simulink model "Ex4_System_Level_AntennaArray"  (R2025b)
settings: Solver=VariableStepDiscrete  StartTime=0.0  StopTime=0.01  RelTol=1e-3
InitFcn:
  | fs         = 8e6;
  | Ts         = 1/fs;
  | fc         = 2.4e9;
  | c          = physconst("LightSpeed");
  | lambda     = freq2wavelen(fc,c);
  | arraySize  = [8,8];
  | targetRCS  = 10.0;
  | targetPosition = [30e3,0,0];
  | targetDist = sqrt(targetPosition(1)^2 + targetPosition(2)^2 + targetPosition(3)^2)
  | pulseWidth = 1e-6;
  | PRF        = 4000;
  | maxRange   = 40e3;
  | 
  | %% Matched filter parameters
  | estimatedDelay = 0; % signal processing delay (in case of buffering)
  | 
  | hwav = phased.RectangularWaveform(...
  |     'PulseWidth',pulseWidth,...
  |     'PRF',PRF,...
  |     'SampleRate',fs);
  | matchingCoeff = getMatchedFilter(hwav);
  | % Delay introduced due to filter
  | matchingDelay = size(matchingCoeff,1)-1;
  | 
  | % Time varying gain parameters
  | fastTimeGrid = unigrid(0,1/fs,1/PRF,'[)');
  | rangeGates = c*fastTimeGrid/2;
  | metersPerSample = rangeGates(2);
  | rangeOffset = -rangeGates(2)*(matchingDelay+estimatedDelay);
  | rangeLoss = 2*fspl(rangeGates,lambda);
  | rangeLoss(1:5) = 0;
  | rangeLoss(end:end-1) = 0;
  | referenceLoss = 2*fspl(maxRange,lambda);
undefined symbols (not defined in the file): physconst
libraries: dspstat3 x10, phasedenvlib x4, phaseddetectlib x3, rfmathmodels2 x2, phasedtxrxlib x2, matrix_library x2, commrflib2 x1, phasedwavlib x1, dspmathops x1
settings Model: Creator=galberti  LastModifiedBy=galberti
settings DebuggingCC: UnderSpecifiedDimensionMsg=warning

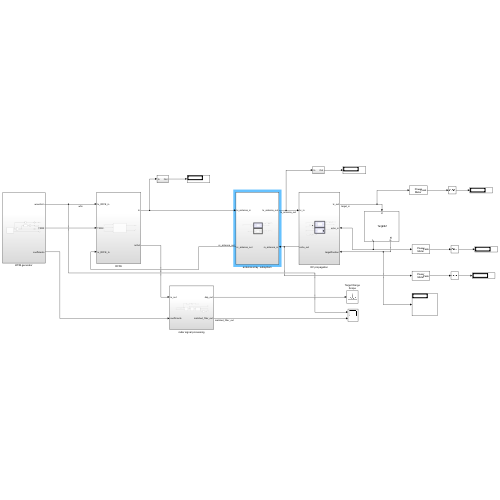
[thumbnail: Simulink's stored preview of the top-level diagram]
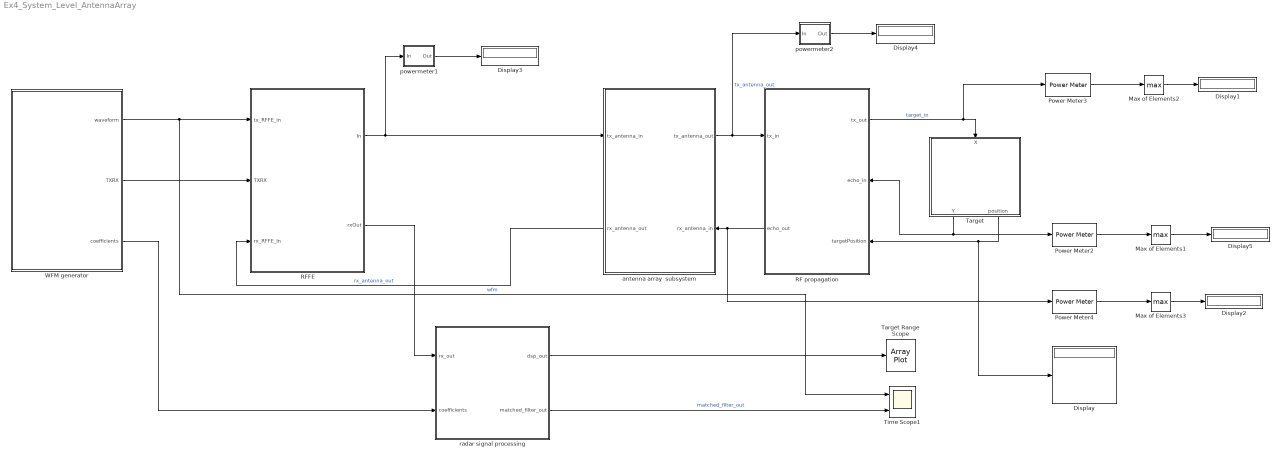
== system Ex4_System_Level_AntennaArray ==
  Display{,1..5} (6 alike) : Display
  Max of Elements1 : MinMax  Function=max
  Max of Elements2 : MinMax  Function=max
  Max of Elements3 : MinMax  Function=max
  Power Meter2 : dspstat3/Power Meter  Measurement=Peak power  ReferenceLoad=1  OutputPowerUnits=dBW  WindowLength=256  OverlapLength=255  AllowArbitraryInputLength=off  ComputeCCDF=off  PowerRange=50  PowerResolution=0.1  CCDFOutput=Relative power (dB above average power)  ProbabilityVector=[ 10; 1; 0.1; 0.01; 0.001; 0.0001 ]  RelativePowerVector=[ 0; 3; 6; 9; 12 ]  ResetPort=off  SimulateUsing=Interpreted execution
  Power Meter3 : dspstat3/Power Meter  Measurement=Peak power  ReferenceLoad=1  OutputPowerUnits=dBW  WindowLength=256  OverlapLength=255  AllowArbitraryInputLength=off  ComputeCCDF=off  PowerRange=50  PowerResolution=0.1  CCDFOutput=Relative power (dB above average power)  ProbabilityVector=[ 10; 1; 0.1; 0.01; 0.001; 0.0001 ]  RelativePowerVector=[ 0; 3; 6; 9; 12 ]  ResetPort=off  SimulateUsing=Interpreted execution
  Power Meter4 : dspstat3/Power Meter  Measurement=Peak power  ReferenceLoad=1  OutputPowerUnits=dBW  WindowLength=256  OverlapLength=255  AllowArbitraryInputLength=off  ComputeCCDF=off  PowerRange=50  PowerResolution=0.1  CCDFOutput=Relative power (dB above average power)  ProbabilityVector=[ 10; 1; 0.1; 0.01; 0.001; 0.0001 ]  RelativePowerVector=[ 0; 3; 6; 9; 12 ]  ResetPort=off  SimulateUsing=Interpreted execution
  RF propagation : Subsystem
      settings: PortSchema="{\"entries\":[{\"content\":{\"sides\":[{\"content\":{\"connectorIds\":[\"In1\",\"Out2\"]},\"type\":\"ConnectorPlacement.EquallySpacedRectSide\",\"uuid\":\"4a1c7530-7650-4dc9-828c-c105decb95b0\"},{\"content\":{\"connectorIds\":[\"Out1\",\"In2\",\"In3\"],\"side\":\"RIGHT\"},\"type\":\"ConnectorPlacement.EquallySpacedRectSide\",\"uuid\":\"d3ec3a06-d85c-4d77-b8ee-6c5e19a3832b\"},{\"content\":{\"side\":\"TOP\"},\"type\":\"ConnectorPlacement.EquallySpacedRectSide\",\"uuid\":\"eb5f04b0-97d0-44f9-917a-0a19ff17b8bd\"}]},\"type\":\"ConnectorPlacement.EquallySpacedConnector\",\"uuid\":\"636c631f-5f34-44d2-af89-1574ca2134a6\"}],\"packageUris\":[\"http://schema.mathworks.com/mf0/Connector/R2020b\"],\"version\":\"1.0\"}"
  RFFE : Subsystem
  Target : Subsystem
      settings: PortSchema="{\"entries\":[{\"content\":{\"sides\":[{\"content\":{},\"type\":\"ConnectorPlacement.EquallySpacedRectSide\",\"uuid\":\"8a6fd2f7-d15e-4a2e-b1e0-7a96b21b95fb\"},{\"content\":{\"side\":\"RIGHT\"},\"type\":\"ConnectorPlacement.EquallySpacedRectSide\",\"uuid\":\"bc3a7d9e-f691-43b7-91d6-b93852d4fa00\"},{\"content\":{\"connectorIds\":[\"In1\"],\"side\":\"TOP\"},\"type\":\"ConnectorPlacement.EquallySpacedRectSide\",\"uuid\":\"7ed9c8d2-fd28-46f2-9526-28705f091796\"},{\"content\":{\"connectorIds\":[\"Out1\",\"Out2\"],\"side\":\"BOTTOM\"},\"type\":\"ConnectorPlacement.EquallySpacedRectSide\",\"uuid\":\"18e6cb2d-6873-45d3-ad7e-d642b2ec4bb6\"}]},\"type\":\"ConnectorPlacement.EquallySpacedConnector\",\"uuid\":\"97cbfb25-2a62-4885-bca6-0491b6cac52b\"}],\"packageUris\":[\"http://schema.mathworks.com/mf0/Connector/R2020b\"],\"version\":\"1.0\"}"
      mask Display:
      | disp('Targets')
      | port_label('input',1,'X');
      | port_label('output',1,'Y');
      | port_label('output',2,'Pos');
      | port_label('output',3,'Vel');
  Target Range Scope : ArrayPlot  WindowPosition=[258.000000,40.000000,765.000000,641.000000,]  Visible=on  ScopeFrameLocation=window  SampleIncrement=metersPerSample  XOffset=rangeOffset  PlotType=Line  AxesScaling=Manual  MaximizeAxes=On  Title=Radar Return  XLabel=Range (m)  YLimits=[-0.0003 0.0026]  ExpandToolstrip=on
  Time Scope1 : Scope  NumInputPorts=2
      settings: TimeUnits=Metric (based on Time Span)  ActiveDisplayYMinimum=-0.0019505702905784962  ActiveDisplayYMaximum=0.0013717401736854759  YLabel=Amplitude
  WFM generator : Subsystem
  antenna array  subsystem : Subsystem
      settings: PortSchema="{\"entries\":[{\"content\":{\"sides\":[{\"content\":{\"connectorIds\":[\"In1\",\"Out2\"]},\"type\":\"ConnectorPlacement.EquallySpacedRectSide\",\"uuid\":\"4a1c7530-7650-4dc9-828c-c105decb95b0\"},{\"content\":{\"connectorIds\":[\"Out1\",\"In2\"],\"side\":\"RIGHT\"},\"type\":\"ConnectorPlacement.EquallySpacedRectSide\",\"uuid\":\"d3ec3a06-d85c-4d77-b8ee-6c5e19a3832b\"},{\"content\":{\"side\":\"TOP\"},\"type\":\"ConnectorPlacement.EquallySpacedRectSide\",\"uuid\":\"eb5f04b0-97d0-44f9-917a-0a19ff17b8bd\"},{\"content\":{\"side\":\"BOTTOM\"},\"type\":\"ConnectorPlacement.EquallySpacedRectSide\",\"uuid\":\"53210fec-ed1a-4dc4-91e9-224cfdf02ee3\"}]},\"type\":\"ConnectorPlacement.EquallySpacedConnector\",\"uuid\":\"636c631f-5f34-44d2-af89-1574ca2134a6\"}],\"packageUris\":[\"http://schema.mathworks.com/mf0/Connector/R2020b\"],\"version\":\"1.0\"}"
  powermeter1 : Subsystem
  powermeter2 : Subsystem
  radar signal processing : Subsystem
  wires:
  WFM generator/1(waveform) -> Time Scope1/1, RFFE/1(tx_RFFE_in)  "wfm"
  WFM generator/3(coefficients) -> radar signal processing/2(coefficients)
  RF propagation/1(tx_out) -> Target/1(X), Power Meter3/1  "target_in"
  antenna array  subsystem/2(rx_antenna_out) -> RFFE/3(rx_RFFE_In)  "rx_antenna_out"
  antenna array  subsystem/1(tx_antenna_out) -> powermeter2/1(In), RF propagation/1(tx_in)  "tx_antenna_out"
  Target/1(Y) -> RF propagation/2(echo_in), Power Meter2/1
  Max of Elements1/1 -> Display5/1
  Power Meter2/1 -> Max of Elements1/1
  radar signal processing/1(dsp_out) -> Target Range Scope/1
  radar signal processing/2(matched_filter_out) -> Time Scope1/2  "matched_filter_out"
  Max of Elements2/1 -> Display1/1
  Power Meter3/1 -> Max of Elements2/1
  RF propagation/2(echo_out) -> Power Meter4/1, antenna array  subsystem/2(rx_antenna_in)
  Max of Elements3/1 -> Display2/1
  Power Meter4/1 -> Max of Elements3/1
  WFM generator/2(TXRX) -> RFFE/2(TXRX)
  RFFE/2(rxOut) -> radar signal processing/1(rx_out)
  RFFE/1(In) -> antenna array  subsystem/1(tx_antenna_in), powermeter1/1(In)
  powermeter1/1(Out) -> Display3/1
  powermeter2/1(Out) -> Display4/1
  Target/2(position) -> Display/1, RF propagation/3(targetPosition)

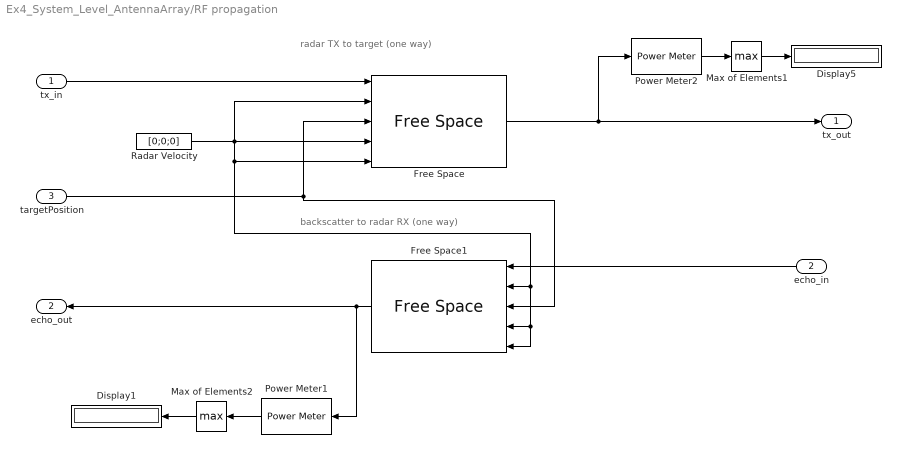
== system Ex4_System_Level_AntennaArray/RF propagation ==
  note: backscatter to radar RX (one way)
  note: radar TX to target (one way)
  tx_in : Inport
  echo_in : Inport  Port=2
  targetPosition : Inport  Port=3
  Display1 : Display
  Display5 : Display
  Free Space : phasedenvlib/Free Space  PropagationSpeed=physconst( 'LightSpeed' )  OperatingFrequency=fc  TwoWayPropagation=off  SampleRateFromInputCheckbox=off  SampleRate=fs  MaximumDistanceSource=Property  MaximumDistance=2*max(targetDist)  MaximumNumInputSamplesSource=Auto  MaximumNumInputSamples=1000  SimulateUsing=Interpreted execution
  Free Space1 : phasedenvlib/Free Space  PropagationSpeed=physconst( 'LightSpeed' )  OperatingFrequency=fc  TwoWayPropagation=off  SampleRateFromInputCheckbox=on  SampleRate=1e6  MaximumDistanceSource=Property  MaximumDistance=2*max(targetDist)  MaximumNumInputSamplesSource=Auto  MaximumNumInputSamples=1000  SimulateUsing=Interpreted execution
  Max of Elements1 : MinMax  Function=max
  Max of Elements2 : MinMax  Function=max
  Power Meter1 : dspstat3/Power Meter  Measurement=Peak power  ReferenceLoad=1  OutputPowerUnits=dBW  WindowLength=256  OverlapLength=255  AllowArbitraryInputLength=off  ComputeCCDF=off  PowerRange=50  PowerResolution=0.1  CCDFOutput=Relative power (dB above average power)  ProbabilityVector=[ 10; 1; 0.1; 0.01; 0.001; 0.0001 ]  RelativePowerVector=[ 0; 3; 6; 9; 12 ]  ResetPort=off  SimulateUsing=Interpreted execution
  Power Meter2 : dspstat3/Power Meter  Measurement=Peak power  ReferenceLoad=1  OutputPowerUnits=dBW  WindowLength=256  OverlapLength=255  AllowArbitraryInputLength=off  ComputeCCDF=off  PowerRange=50  PowerResolution=0.1  CCDFOutput=Relative power (dB above average power)  ProbabilityVector=[ 10; 1; 0.1; 0.01; 0.001; 0.0001 ]  RelativePowerVector=[ 0; 3; 6; 9; 12 ]  ResetPort=off  SimulateUsing=Interpreted execution
  Radar Velocity : Constant  Value=[0;0;0]  SampleTime=-1
  tx_out : Outport
  echo_out : Outport  Port=2
  wires:
  tx_in/1 -> Free Space/1
  Free Space1/1 -> echo_out/1, Power Meter1/1
  Free Space/1 -> Power Meter2/1, tx_out/1
  echo_in/1 -> Free Space1/1
  Radar Velocity/1 -> Free Space/5, Free Space1/5, Free Space1/4, Free Space1/2, Free Space/2, Free Space/4
  targetPosition/1 -> Free Space1/3, Free Space/3
  Power Meter2/1 -> Max of Elements1/1
  Max of Elements1/1 -> Display5/1
  Power Meter1/1 -> Max of Elements2/1
  Max of Elements2/1 -> Display1/1

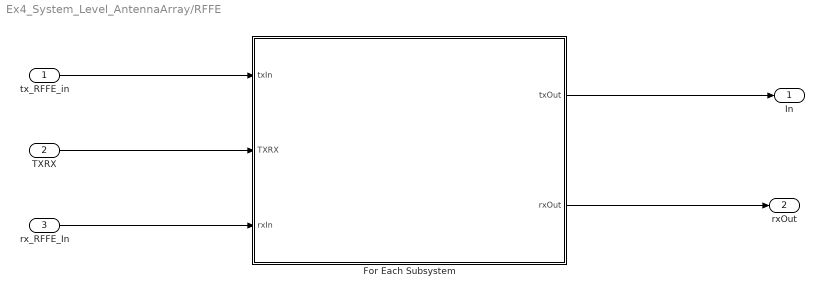
== system Ex4_System_Level_AntennaArray/RFFE ==
  tx_RFFE_in : Inport
  TXRX : Inport  Port=2
  rx_RFFE_In : Inport  Port=3
  For Each Subsystem : Subsystem  TreatAsAtomicUnit=on
  In : Outport
  rxOut : Outport  Port=2
  wires:
  tx_RFFE_in/1 -> For Each Subsystem/1(txIn)
  TXRX/1 -> For Each Subsystem/2(TXRX)
  For Each Subsystem/1(txOut) -> In/1
  rx_RFFE_In/1 -> For Each Subsystem/3(rxIn)
  For Each Subsystem/2(rxOut) -> rxOut/1

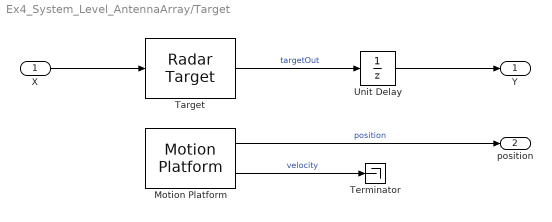
== system Ex4_System_Level_AntennaArray/Target ==
  X : Inport
  Motion Platform : phasedenvlib/Motion Platform  MotionModel=Velocity  InitialPosition=targetPosition'  InitialVelocity=[ 0; 0; 0 ]  VelocitySource=Property  Velocity=[0;0;0]  AccelerationSource=Property  Acceleration=[0;0;0]  CustomTrajectory=[ 0, 0, 0, 0, 0, 0, 0; 1, 0, 0, 0, 0, 0, 0 ]  ScanMode=None  InitialScanAngle=0  AzimuthSpan=[ -60, 60 ]  AzimuthScanRate=10  InitialOrientationAxes=eye(3)  OrientationAxesOutputPort=off  ElapsedTimeSource=Auto  SampleRateFromInputCheckbox=on  SampleRate=1e6  SimulateUsing=Interpreted execution
  Target : phasedenvlib/Radar Target  EnablePolarization=off  Mode=Monostatic  MeanRCSSource=Property  ScatteringMatrixSource=Property  MeanRCS=targetRCS  ScatteringMatrix=eye( 2 )  Model=Nonfluctuating  PropagationSpeed=physconst('LightSpeed')  OperatingFrequency=fc  SeedSource=Auto  Seed=0  SimulateUsing=Interpreted execution
  Terminator : Terminator
  Unit Delay : UnitDelay  SampleTime=-1  HasFrameUpgradeWarning=on
  Y : Outport  VectorParamsAs1DForOutWhenUnconnected=off
  position : Outport  Port=2  VectorParamsAs1DForOutWhenUnconnected=off
  wires:
  X/1 -> Target/1
  Target/1 -> Unit Delay/1  "targetOut"
  Unit Delay/1 -> Y/1
  Motion Platform/2 -> Terminator/1  "velocity"
  Motion Platform/1 -> position/1  "position"

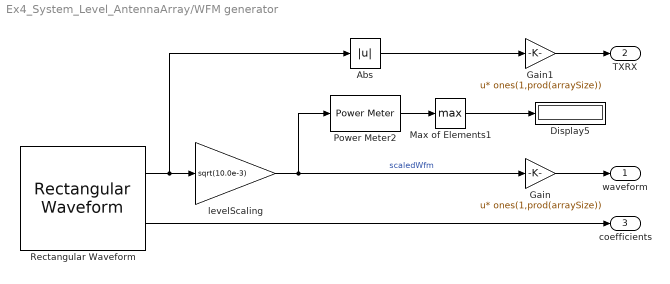
== system Ex4_System_Level_AntennaArray/WFM generator ==
  Abs : Abs  SaturateOnIntegerOverflow=off
  Display5 : Display
  Gain : Gain  Gain=ones(1,prod(arraySize))  Multiplication=Matrix(u*K)
  Gain1 : Gain  Gain=ones(1,prod(arraySize))  Multiplication=Matrix(u*K)
  Max of Elements1 : MinMax  Function=max
  Power Meter2 : dspstat3/Power Meter  Measurement=Peak power  ReferenceLoad=1  OutputPowerUnits=dBW  WindowLength=256  OverlapLength=255  AllowArbitraryInputLength=off  ComputeCCDF=off  PowerRange=50  PowerResolution=0.1  CCDFOutput=Relative power (dB above average power)  ProbabilityVector=[ 10; 1; 0.1; 0.01; 0.001; 0.0001 ]  RelativePowerVector=[ 0; 3; 6; 9; 12 ]  ResetPort=off  SimulateUsing=Interpreted execution
  Rectangular Waveform : phasedwavlib/Rectangular Waveform  SampleRate=fs  DurationSpecification=Pulse width  PulseWidth=pulseWidth  DutyCycle=0.5  PRF=PRF  PRFSelectionInputPort=off  SimulationTimeSource=Derive from waveform parameters  FrequencyOffsetSource=Property  FrequencyOffset=0  OutputFormat=Pulses  NumSamples=100  NumPulses=1  PRFOutputPort=off  CoefficientsOutputPort=on  SimulateUsing=Interpreted execution
  levelScaling : Gain  Gain=sqrt(10.0e-3)
  waveform : Outport
  TXRX : Outport  Port=2
  coefficients : Outport  Port=3
  wires:
  Rectangular Waveform/2 -> coefficients/1
  Rectangular Waveform/1 -> Abs/1, levelScaling/1
  levelScaling/1 -> Power Meter2/1, Gain/1  "scaledWfm"
  Abs/1 -> Gain1/1
  Power Meter2/1 -> Max of Elements1/1
  Max of Elements1/1 -> Display5/1
  Gain/1 -> waveform/1
  Gain1/1 -> TXRX/1

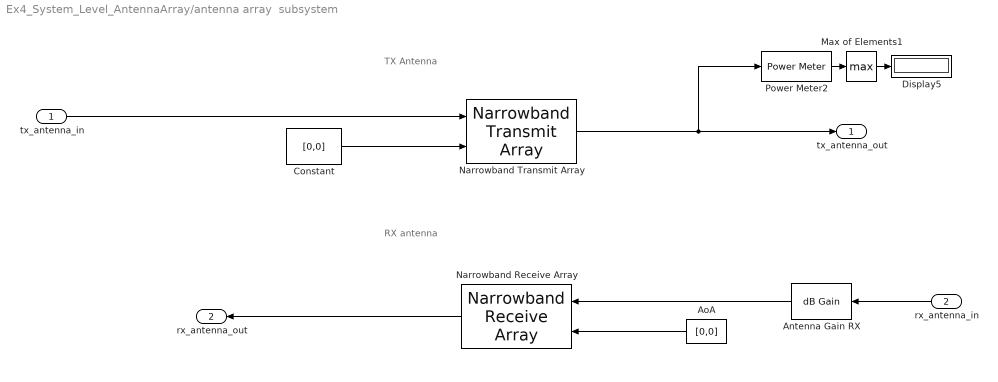
== system Ex4_System_Level_AntennaArray/antenna array  subsystem ==
  note: RX antenna
  note: TX Antenna
  tx_antenna_in : Inport
  rx_antenna_in : Inport  Port=2
  Antenna Gain RX : dspmathops/dB Gain  dB=7  intype=Amplitude
  AoA : Constant  Value=[0,0]
  Constant : Constant  Value=[0,0]
  Display5 : Display
  Max of Elements1 : MinMax  Function=max
  Narrowband Receive Array : phasedtxrxlib/Narrowband Receive Array  PropagationSpeed=physconst( 'LightSpeed' )  OperatingFrequency=fc  Wavefront=Plane  SensorGainMeasure=dBi  Polarization=None  WeightsInputPort=off  SimulateUsing=Interpreted execution  Sensor=phased.URA(Size=arraySize,ElementSpacing=[ 0.5, 0.5 ].*lambda,ArrayNormal='x',Element=phased.IsotropicAntennaElement())
  Narrowband Transmit Array : phasedtxrxlib/Narrowband Transmit Array  PropagationSpeed=physconst( 'LightSpeed' )  OperatingFrequency=fc  CombineRadiatedSignals=on  SensorGainMeasure=dB  Polarization=None  WeightsInputPort=off  SimulateUsing=Interpreted execution  Sensor=phased.URA(Size=arraySize,ElementSpacing=[ 0.5, 0.5 ].*lambda,Lattice='Triangular',ArrayNormal='x',Element=phased.IsotropicAntennaElement(BackBaffled=true))
  Power Meter2 : dspstat3/Power Meter  Measurement=Peak power  ReferenceLoad=1  OutputPowerUnits=dBW  WindowLength=256  OverlapLength=255  AllowArbitraryInputLength=off  ComputeCCDF=off  PowerRange=50  PowerResolution=0.1  CCDFOutput=Relative power (dB above average power)  ProbabilityVector=[ 10; 1; 0.1; 0.01; 0.001; 0.0001 ]  RelativePowerVector=[ 0; 3; 6; 9; 12 ]  ResetPort=off  SimulateUsing=Interpreted execution
  tx_antenna_out : Outport
  rx_antenna_out : Outport  Port=2
  wires:
  Constant/1 -> Narrowband Transmit Array/2
  Narrowband Receive Array/1 -> rx_antenna_out/1
  rx_antenna_in/1 -> Antenna Gain RX/1
  Narrowband Transmit Array/1 -> Power Meter2/1, tx_antenna_out/1
  AoA/1 -> Narrowband Receive Array/2
  Power Meter2/1 -> Max of Elements1/1
  Max of Elements1/1 -> Display5/1
  tx_antenna_in/1 -> Narrowband Transmit Array/1
  Antenna Gain RX/1 -> Narrowband Receive Array/1

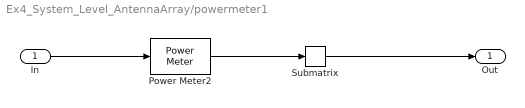
== system Ex4_System_Level_AntennaArray/powermeter1 ==
  In : Inport
  Power Meter2 : dspstat3/Power Meter  Measurement=Peak power  ReferenceLoad=1  OutputPowerUnits=dBW  WindowLength=fs/PRF  OverlapLength=fs/PRF-1  AllowArbitraryInputLength=off  ComputeCCDF=off  PowerRange=50  PowerResolution=0.1  CCDFOutput=Relative power (dB above average power)  ProbabilityVector=[ 10; 1; 0.1; 0.01; 0.001; 0.0001 ]  RelativePowerVector=[ 0; 3; 6; 9; 12 ]  ResetPort=off  SimulateUsing=Interpreted execution
      settings: LibrarySourceBlock=commutil2/Power Meter
  Submatrix : matrix_library/Submatrix  RowSpan=One row  RowStartMode=Last  RowStartIndex=1  RowEndMode=Index  RowEndIndex=Ndist  ColSpan=One column  ColStartMode=Last  ColStartIndex=1  ColEndMode=Last  ColEndIndex=1
  Out : Outport
  wires:
  In/1 -> Power Meter2/1
  Submatrix/1 -> Out/1
  Power Meter2/1 -> Submatrix/1

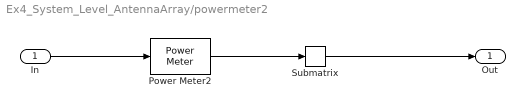
== system Ex4_System_Level_AntennaArray/powermeter2 ==
  In : Inport
  Power Meter2 : dspstat3/Power Meter  Measurement=Peak power  ReferenceLoad=1  OutputPowerUnits=dBW  WindowLength=fs/PRF  OverlapLength=fs/PRF-1  AllowArbitraryInputLength=off  ComputeCCDF=off  PowerRange=50  PowerResolution=0.1  CCDFOutput=Relative power (dB above average power)  ProbabilityVector=[ 10; 1; 0.1; 0.01; 0.001; 0.0001 ]  RelativePowerVector=[ 0; 3; 6; 9; 12 ]  ResetPort=off  SimulateUsing=Interpreted execution
      settings: LibrarySourceBlock=commutil2/Power Meter
  Submatrix : matrix_library/Submatrix  RowSpan=One row  RowStartMode=Last  RowStartIndex=1  RowEndMode=Index  RowEndIndex=Ndist  ColSpan=One column  ColStartMode=Last  ColStartIndex=1  ColEndMode=Last  ColEndIndex=1
  Out : Outport
  wires:
  In/1 -> Power Meter2/1
  Submatrix/1 -> Out/1
  Power Meter2/1 -> Submatrix/1

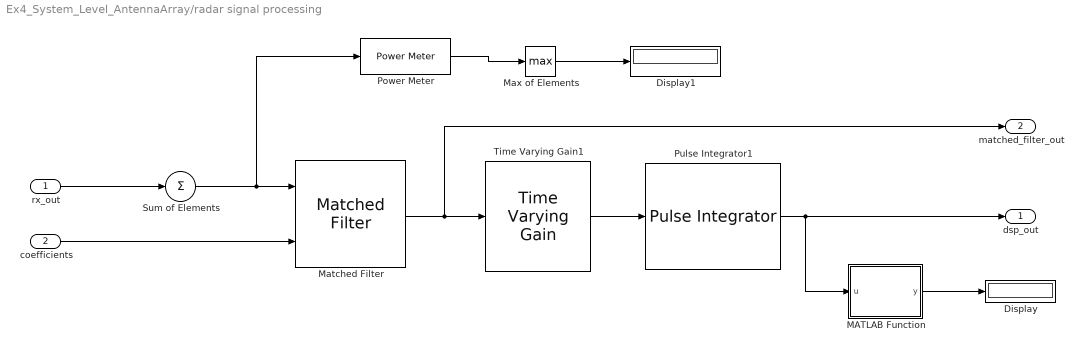
== system Ex4_System_Level_AntennaArray/radar signal processing ==
  rx_out : Inport
  coefficients : Inport  Port=2
  Display : Display
  Display1 : Display
  MATLAB Function : MATLAB Function  TreatAsAtomicUnit=on
  Matched Filter : phaseddetectlib/Matched Filter  CoefficientsSource=Input port  Coefficients=[ 1; 1 ]  SpectrumWindow=None  CustomSpectrumWindow=@hamming  SpectrumRange=[ 0, 1e5 ]  SampleRateFromInputCheckbox=on  SampleRate=1e6  SidelobeAttenuation=30  Beta=0.5  Nbar=4  GainOutputPort=off  MaximumNumInputSamplesSource=Auto  MaximumNumInputSamples=100  SimulateUsing=Interpreted execution
  Max of Elements : MinMax  Function=max
  Power Meter : dspstat3/Power Meter  Measurement=Peak power  ReferenceLoad=1  OutputPowerUnits=dBW  WindowLength=256  OverlapLength=255  AllowArbitraryInputLength=off  ComputeCCDF=off  PowerRange=50  PowerResolution=0.1  CCDFOutput=Relative power (dB above average power)  ProbabilityVector=[ 10; 1; 0.1; 0.01; 0.001; 0.0001 ]  RelativePowerVector=[ 0; 3; 6; 9; 12 ]  ResetPort=off  SimulateUsing=Interpreted execution
  Pulse Integrator1 : phaseddetectlib/Pulse Integrator  CoherentFlag=Noncoherent  N=10  V=9
  Sum of Elements : Sum  Inputs=+  CollapseMode=Specified dimension  CollapseDim=2
  Time Varying Gain1 : phaseddetectlib/Time Varying Gain  RangeLossSource=Property  RangeLoss=rangeLoss  ReferenceLoss=referenceLoss  SimulateUsing=Interpreted execution
  dsp_out : Outport
  matched_filter_out : Outport  Port=2
  wires:
  rx_out/1 -> Sum of Elements/1
  Pulse Integrator1/1 -> MATLAB Function/1(u), dsp_out/1
  Matched Filter/1 -> matched_filter_out/1, Time Varying Gain1/1
  Time Varying Gain1/1 -> Pulse Integrator1/1
  coefficients/1 -> Matched Filter/2
  MATLAB Function/1(y) -> Display/1
  Sum of Elements/1 -> Power Meter/1, Matched Filter/1
  Power Meter/1 -> Max of Elements/1
  Max of Elements/1 -> Display1/1

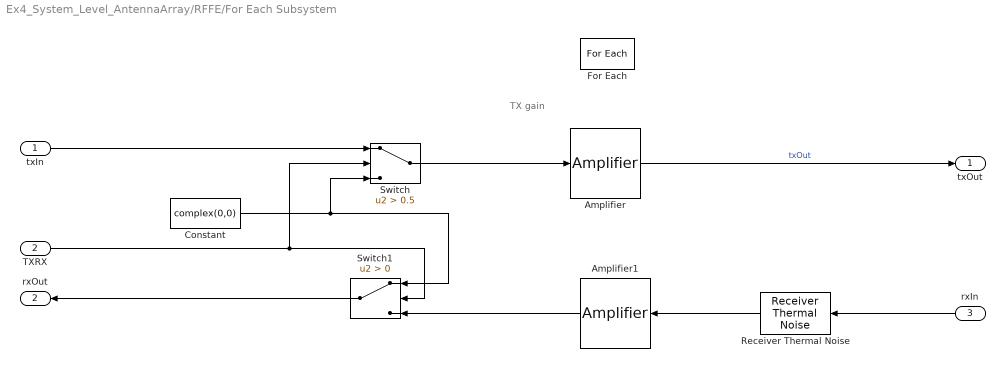
== system Ex4_System_Level_AntennaArray/RFFE/For Each Subsystem ==
  note: TX gain
  txIn : Inport  Partition=on  PartitionDimension=2  PartitionWidth=1  PartitionOffset=0
  TXRX : Inport  Port=2  Partition=on  PartitionDimension=2  PartitionWidth=1  PartitionOffset=0
  rxIn : Inport  Port=3  Partition=on  PartitionDimension=2  PartitionWidth=1  PartitionOffset=0
  Amplifier : rfmathmodels2/Amplifier  Model=cubic  Gain=55  Nonlinearity=OIP3  IIP3=Inf  OIP3=Inf  IP1dB=Inf  OP1dB=Inf  IPsat=Inf  OPsat=Inf  Table=[ -25, 5, -1; -10, 20, -2; 0, 27, 5; 5, 28, 12 ]  MagnitudeGainDB=0  Vsat=1  MagnitudeSmooth=2  PhaseGainRadian=-.45  PhaseSaturation=.88  PhaseSmooth=[ 3.43, 3.43 ]  InputScaleDB=0  AmAmParameters=[ 2.1587, 1.1517 ]  AmPmParameters=[ 4.0033, 9.1040 ]  OutputScaleDB=0  SimulateUsing=Interpreted execution  IncludeNoise=off  NoiseType=NF  NoiseTemperature=290  NF=3  NoiseFactor=2  SeedSource=auto  Seed=67987  SampleRate=1e6
  Amplifier1 : rfmathmodels2/Amplifier  Model=cubic  Gain=39  Nonlinearity=OIP3  IIP3=Inf  OIP3=Inf  IP1dB=Inf  OP1dB=Inf  IPsat=Inf  OPsat=Inf  Table=[ -25, 5, -1; -10, 20, -2; 0, 27, 5; 5, 28, 12 ]  MagnitudeGainDB=0  Vsat=1  MagnitudeSmooth=2  PhaseGainRadian=-.45  PhaseSaturation=.88  PhaseSmooth=[ 3.43, 3.43 ]  InputScaleDB=0  AmAmParameters=[ 2.1587, 1.1517 ]  AmPmParameters=[ 4.0033, 9.1040 ]  OutputScaleDB=0  SimulateUsing=Interpreted execution  IncludeNoise=off  NoiseType=NF  NoiseTemperature=290  NF=6  NoiseFactor=2  SeedSource=auto  Seed=67987  SampleRate=1e6
  Constant : Constant  Value=complex(0,0)
  For Each : ForEach  DisableCoverage=on
  Receiver Thermal Noise : commrflib2/Receiver Thermal Noise  LegacyMode=off  NoiseMethod=Noise temperature  NoiseTemperature=290  NoiseFigure=3.0103  NoiseFactor=2  Add290KAntennaNoise=off  ReferenceLoad=1  RandomStream=Global stream  Seed=floor(rand(1,1)*1000)  SimulateUsing=Interpreted execution
  Switch : Switch  Criteria=u2 > Threshold  Threshold=0.5  SaturateOnIntegerOverflow=off  InputSameDT=off
  Switch1 : Switch  Criteria=u2 > Threshold  SaturateOnIntegerOverflow=off  InputSameDT=off
  txOut : Outport  ConcatenationDimension=2
  rxOut : Outport  Port=2  ConcatenationDimension=2
  wires:
  txIn/1 -> Switch/1
  Amplifier1/1 -> Switch1/3
  Receiver Thermal Noise/1 -> Amplifier1/1
  Switch/1 -> Amplifier/1
  TXRX/1 -> Switch/2, Switch1/2
  Amplifier/1 -> txOut/1  "txOut"
  Constant/1 -> Switch/3, Switch1/1
  rxIn/1 -> Receiver Thermal Noise/1
  Switch1/1 -> rxOut/1

== matlab function Ex4_System_Level_AntennaArray/radar signal processing/MATLAB Function ==
  data: u input; y output; metersPerSample parameter; rangeOffset parameter
function y = targetDistance(u, metersPerSample, rangeOffset)
[~,idx] = max(u);
N=length(u);
distance = (0:N-1)*metersPerSample+rangeOffset;
y = distance(idx)/1e3;
